simulink model "case 4"  (R2018a)
settings: Solver=VariableStepAuto  StartTime=0.0  StopTime=6  RelTol=1e-3
values from neighbouring files (symbols this model uses):
  cdcc = 0.00022    [matlab.mat]
  cf = 8e-05    [matlab.mat]
  iodmax = 12    [matlab.mat]
  iqdmax = -7.2    [matlab.mat]
  kiid = 0.5    [matlab.mat]
  kiiq = -5    [matlab.mat]
  kpid = 0.4    [matlab.mat]
  kpiq = -4    [matlab.mat]
  lf = 0.0075    [matlab.mat]
  ll = 1e-06    [matlab.mat]
  md = 0.001    [matlab.mat]
  nq = 0.002    [matlab.mat]
  p0 = 240    [matlab.mat]
  q0 = 60    [matlab.mat]
  rf = 0.0015    [matlab.mat]
  rl = 0.001    [matlab.mat]
  vdc = 200    [matlab.mat]
  wc = 0.000125663706144    [matlab.mat]
undefined symbols (not defined in the file or in its folder): DiscIntNeverNeededParam, gcbh, sps, sps_rtmsupport
libraries: powerlib_meascontrol x31, neural x30, powerlib x23, spsVIMeasurementModel x6, simulink x4
(part 3 of 3)

== system case 4/Controller/NN Controller1/Function Fitting Neural Network/Layer 2/LW{2,1} ==
  "ad{2,1}" : Inport  PortDimensions=10
      mask Display: e = 0.06;c1 = [120 230 180]/255;c2 = ([120 230 180]+0)/(256+128);c3 = ([120 230 180]+128)/(256+128);patch([0 1 1 0],[0 0 1 1],c1);patch([0 1 1 1-e 1-e 0+e],[0 0 1 1-e 0+e 0+e],c2);patch([0 0 1 1-e 0+e 0+e],[0 1 1 1-e 1-e 0+e],c3);plot([0 1 1 0 0],[0 0 1 1 0]);
  "IW{2,1}(1,:)'" : Constant  Value=[-0.1816600740664736923779543076307163573801517486572265625;0.1840405874166839428340836093411780893802642822265625;-0.0692395627232279819995852676584036089479923248291015625;0.0661828291573189619878547773623722605407238006591796875;0.055642219905920546618727229315481963567435741424560546875;-0.052714676109248702340348557981997146271169185638427734375;-0.07678590828023341974262194753464427776634693145751953125;0.054752717540238061977309058647733763791620731353759765625;-0.039136060349110261824545631270666490308940410614013671875;0.219645642177739242040246381293400190770626068115234375]
      mask Display: e = 0.06;c1 = [120 150 230]/255;c2 = ([120 150 230]+0)/383;c3 = ([120 150 230]+128)/383;patch([0 1 1 0],[0 0 1 1],c1);patch([0 1 1 1-e 1-e 0+e],[0 0 1 1-e 0+e 0+e],c2);patch([0 0 1 1-e 0+e 0+e],[0 1 1 1-e 1-e 0+e],c3);plot([0 1 1 0 0],[0 0 1 1 0]);disp('weights');
  Mux : Mux  Inputs=1
      mask Display: e = 0.06;c1 = [120 150 230]/255;c2 = ([120 150 230]+0)/383;c3 = ([120 150 230]+128)/383;patch([0 1 1 0],[0 0 1 1],c1);patch([0 1 1 1-e 1-e 0+e],[0 0 1 1-e 0+e 0+e],c2);patch([0 0 1 1-e 0+e 0+e],[0 1 1 1-e 1-e 0+e],c3);plot([0 1 1 0 0],[0 0 1 1 0]);disp('Mux');
  dotprod1 : neural/Weight Functions/dotprod
  "lz{2,1}" : Outport
      mask Display: e = 0.06;c1 = [120 230 180]/255;c2 = ([120 230 180]+0)/(256+128);c3 = ([120 230 180]+128)/(256+128);patch([0 1 1 0],[0 0 1 1],c1);patch([0 1 1 1-e 1-e 0+e],[0 0 1 1-e 0+e 0+e],c2);patch([0 0 1 1-e 0+e 0+e],[0 1 1 1-e 1-e 0+e],c3);plot([0 1 1 0 0],[0 0 1 1 0]);
  wires:
  "IW{2,1}(1,:)'"/1 -> dotprod1/1
  "ad{2,1}"/1 -> dotprod1/2
  dotprod1/1 -> Mux/1
  Mux/1 -> "lz{2,1}"/1

== system case 4/Controller/RMS4/Mean1/Model/Subsystem ==
  In1 : Inport
  Add : Sum
  Clock : Clock
  Gain1 : Gain  Gain=30/38
  Look-Up Table : Lookup  InputValues=[0 2 2.01 6]  Table=[-0.01 -0.01 -8 -8]  SaturateOnIntegerOverflow=on
  Scope{,1..4} (5 alike) : Scope
  Second-Order Filter : powerlib_meascontrol/Filters/Second-Order Filter  FilterType=Lowpass  Fo=10  Zeta=0.909  Ts=50e-6  Initialize=off  Vac_Init="[0,  0,  60]"  Vdc_Init=0  PlotResponse=off  FreqRange=[0, 500, 1]
      settings: SourceProductName=Simscape Power Systems  SourceProductBaseCode=PS
  Switch : Switch  Criteria=u2 > Threshold
  Uniform Random Number : UniformRandomNumber  Minimum=-0.1  Maximum=0.1  SampleTime=50e-6
  Out1 : Outport
  wires:
  Clock/1 -> Look-Up Table/1
  Look-Up Table/1 -> Second-Order Filter/1
  In1/1 -> Switch/2, Scope/1
  Second-Order Filter/1 -> Switch/1, Switch/3, Scope3/1
  Switch/1 -> Add/1, Scope1/1
  Add/1 -> Scope4/1, Out1/1
  Uniform Random Number/1 -> Add/2
